simulink library "uavsimBlockset_Environment_calmAtmosphere"  (Simulink 8.6)
settings: Solver=ode45  StartTime=0.0  StopTime=10.0  RelTol=1e-3
settings Model: Creator=mstolle  LastModifiedBy=j.bolting

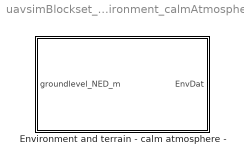
== system uavsimBlockset_Environment_calmAtmosphere ==
  Environment and terrain - calm atmosphere - : Subsystem

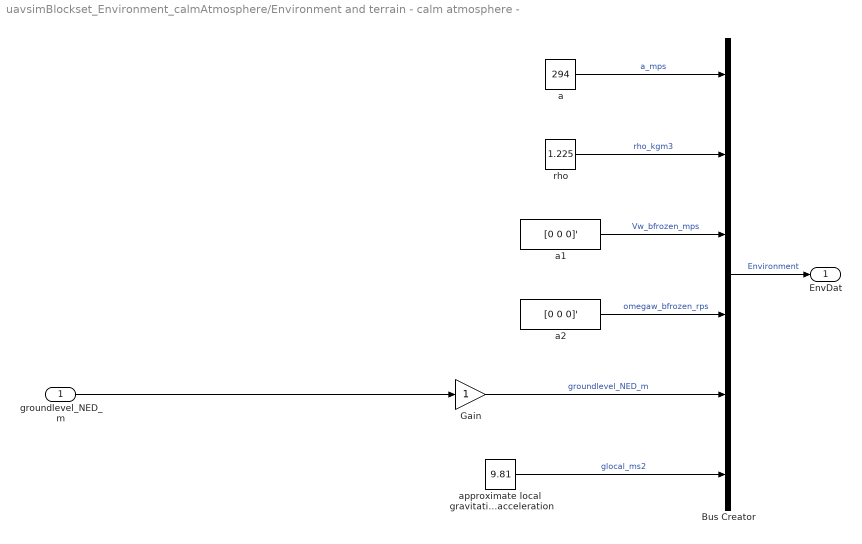
== system uavsimBlockset_Environment_calmAtmosphere/Environment and terrain - calm atmosphere - ==
  groundlevel_NED_m : Inport
  Bus Creator : BusCreator  Inputs=6  OutDataTypeStr=Bus: Environment  NonVirtualBus=on
  Gain : Gain
  a : Constant  Value=294
  a1 : Constant  Value=[0 0 0]'
  a2 : Constant  Value=[0 0 0]'
  approximate local  gravitational acceleration : Constant  Value=9.81
  "rho " : Constant  Value=1.225
  EnvDat : Outport  OutDataTypeStr=Bus: Environment
  wires:
  groundlevel_NED_m/1 -> Gain/1
  Bus Creator/1 -> EnvDat/1  "Environment"
  "rho "/1 -> Bus Creator/2  "rho_kgm3"
  a/1 -> Bus Creator/1  "a_mps"
  a1/1 -> Bus Creator/3  "Vw_bfrozen_mps"
  approximate local  gravitational acceleration/1 -> Bus Creator/6  "glocal_ms2"
  a2/1 -> Bus Creator/4  "omegaw_bfrozen_rps"
  Gain/1 -> Bus Creator/5  "groundlevel_NED_m"
